simulink model "downsample_upsample_example_org"  (Simulink 10.0)
settings: Solver=FixedStepDiscrete  StartTime=0.0  StopTime=10  RelTol=1e-3
libraries: dspsigops x4
settings Model: Creator=svanbeek  LastModifiedBy=annonymous
settings DataIOCC: LimitDataPoints=on  SaveOutput=off  SignalLogging=off  SaveTime=off
settings OptimizationCC: BlockReduction=off  ConditionallyExecuteInputs=off  DefaultParameterBehavior=Inlined  ExpressionDepthLimit=2147483647
settings DebuggingCC: AlgebraicLoopMsg=error  SolverPrmCheckMsg=warning  SingleTaskRateTransMsg=error  StateNameClashWarn=warning
settings HardwareCC: ProdHWDeviceType=ASIC/FPGA->ASIC/FPGA  ProdEqTarget=off
settings GRTTargetCC: GeneratePreprocessorConditionals=Disable all  CombineOutputUpdateFcns=on  GRTInterface=off
settings ConfigComp: CovExternalEMLEnable=off

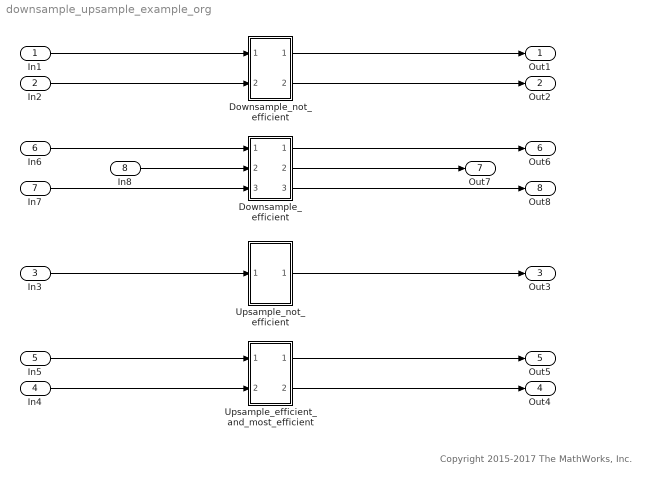
== system downsample_upsample_example_org ==
  note: Copyright 2015-2017 The MathWorks, Inc.
  In1 : Inport  OutDataTypeStr=fixdt(1,16,14)  SampleTime=1
  In2 : Inport  Port=2  OutDataTypeStr=fixdt(1,16,14)  SampleTime=1
  In3 : Inport  Port=3  OutDataTypeStr=fixdt(1,16,14)  SampleTime=1
  In4 : Inport  Port=4  OutDataTypeStr=fixdt(1,16,14)  SampleTime=1
  In5 : Inport  Port=5  OutDataTypeStr=fixdt(1,16,14)  SampleTime=1
  In6 : Inport  Port=6  OutDataTypeStr=fixdt(1,16,14)  SampleTime=1
  In7 : Inport  Port=7  OutDataTypeStr=fixdt(1,16,14)  SampleTime=1
  In8 : Inport  Port=8  OutDataTypeStr=fixdt(1,16,14)  SampleTime=1
  Downsample_efficient : Subsystem
  Downsample_not_efficient : Subsystem
  Upsample_efficient_and_most_efficient : Subsystem
  Upsample_not_efficient : Subsystem
  Out1 : Outport
  Out2 : Outport  Port=2
  Out3 : Outport  Port=3
  Out4 : Outport  Port=4
  Out5 : Outport  Port=5
  Out6 : Outport  Port=6
  Out7 : Outport  Port=7
  Out8 : Outport  Port=8
  wires:
  In1/1 -> Downsample_not_efficient/1(In1)
  In2/1 -> Downsample_not_efficient/2(In2)
  Downsample_not_efficient/1(Out1) -> Out1/1
  Downsample_not_efficient/2(Out2) -> Out2/1
  In3/1 -> Upsample_not_efficient/1(In1)
  In4/1 -> Upsample_efficient_and_most_efficient/2(In2)
  Upsample_not_efficient/1(Out1) -> Out3/1
  Upsample_efficient_and_most_efficient/2(Out2) -> Out4/1
  In5/1 -> Upsample_efficient_and_most_efficient/1(In1)
  Upsample_efficient_and_most_efficient/1(Out1) -> Out5/1
  In6/1 -> Downsample_efficient/1(In1)
  In7/1 -> Downsample_efficient/3(In2)
  Downsample_efficient/1(Out1) -> Out6/1
  Downsample_efficient/2(Out2) -> Out7/1
  In8/1 -> Downsample_efficient/2(In3)
  Downsample_efficient/3(Out3) -> Out8/1

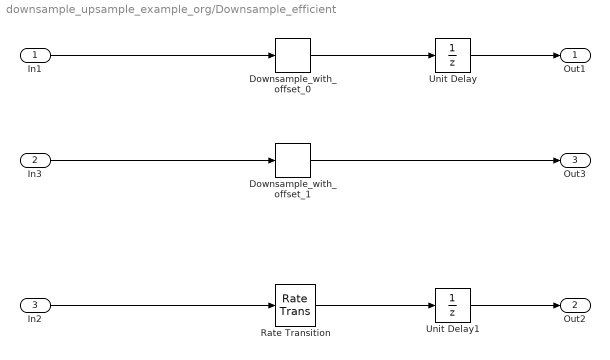
== system downsample_upsample_example_org/Downsample_efficient ==
  In1 : Inport
  In3 : Inport  Port=2
  In2 : Inport  Port=3
  Downsample_with_offset_0 : dspsigops/Downsample  Description=efficient usage of downsample  N=2  phase=0  RateOptions=Allow multirate processing  smode=Allow multirate  fmode=Maintain input frame size  ic=0
      settings: AttributesFormatString=%<Description>  SourceProductName=DSP System Toolbox  SourceProductBaseCode=DS
  Downsample_with_offset_1 : dspsigops/Downsample  Description=|  N=2  phase=1  RateOptions=Allow multirate processing  smode=Allow multirate  fmode=Maintain input frame size  ic=0
      | efficient usage of downsample                                    
      | offset is equal to K-1 eliminates the need for the extra register
      settings: AttributesFormatString=%<Description>  SourceProductName=DSP System Toolbox  SourceProductBaseCode=DS
  Rate Transition : RateTransition  Description=|  OutPortSampleTimeOpt=Multiple of input port sample time  OutPortSampleTimeMultiple=2
      | efficient usage of rate transition
      | similar to downsample
      settings: AttributesFormatString=%<Description>
  Unit Delay : UnitDelay  SampleTime=-1  HasFrameUpgradeWarning=on
  Unit Delay1 : UnitDelay  SampleTime=-1  HasFrameUpgradeWarning=on
  Out1 : Outport
  Out2 : Outport  Port=2
  Out3 : Outport  Port=3
  wires:
  Rate Transition/1 -> Unit Delay1/1
  In2/1 -> Rate Transition/1
  In1/1 -> Downsample_with_offset_0/1
  Downsample_with_offset_0/1 -> Unit Delay/1
  Unit Delay/1 -> Out1/1
  Unit Delay1/1 -> Out2/1
  In3/1 -> Downsample_with_offset_1/1
  Downsample_with_offset_1/1 -> Out3/1

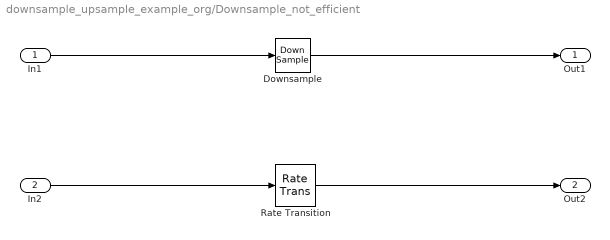
== system downsample_upsample_example_org/Downsample_not_efficient ==
  In1 : Inport
  In2 : Inport  Port=2
  Downsample : DownSample  Description=|  RateOptions=Allow multirate processing
      | inefficient implementation of downsample  
      | requires bypass register and mux          
      | path from input to output is combinatorial
      settings: AttributesFormatString=%<Description>
  Rate Transition : RateTransition  Description=|  OutPortSampleTimeOpt=Multiple of input port sample time  OutPortSampleTimeMultiple=2
      | inefficient implementation of downsample  
      | requires bypass register and mux          
      | path from input to output is combinatorial
      settings: AttributesFormatString=%<Description>
  Out1 : Outport
  Out2 : Outport  Port=2
  wires:
  Downsample/1 -> Out1/1
  In1/1 -> Downsample/1
  In2/1 -> Rate Transition/1
  Rate Transition/1 -> Out2/1

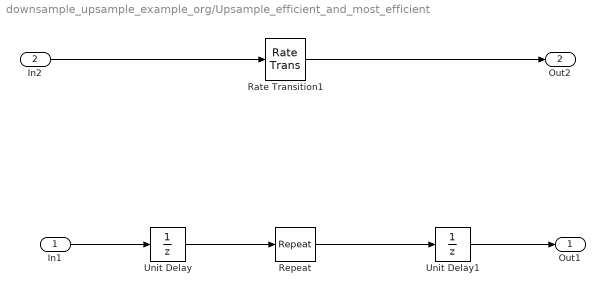
== system downsample_upsample_example_org/Upsample_efficient_and_most_efficient ==
  In1 : Inport
  In2 : Inport  Port=2
  Rate Transition1 : RateTransition  Description=this is an efficient upsample
      settings: AttributesFormatString=%<Description>
  Repeat : dspsigops/Repeat  Description=this becomes just a wire  N=3  RateOptions=Allow multirate processing  ic=0  mode=Unused parameter value
      settings: AttributesFormatString=%<Description>  SourceProductName=DSP System Toolbox
  Unit Delay : UnitDelay  SampleTime=-1  HasFrameUpgradeWarning=on
  Unit Delay1 : UnitDelay  SampleTime=-1  HasFrameUpgradeWarning=on
  Out1 : Outport
  Out2 : Outport  Port=2
  wires:
  Repeat/1 -> Unit Delay1/1
  In1/1 -> Unit Delay/1
  In2/1 -> Rate Transition1/1
  Rate Transition1/1 -> Out2/1
  Unit Delay/1 -> Repeat/1
  Unit Delay1/1 -> Out1/1

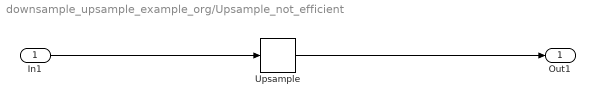
== system downsample_upsample_example_org/Upsample_not_efficient ==
  In1 : Inport
  Upsample : dspsigops/Upsample  N=3  phase=0  RateOptions=Allow multirate processing  ic=0  mode=Unused parameter value
  Out1 : Outport
  wires:
  In1/1 -> Upsample/1
  Upsample/1 -> Out1/1
